simulink model "MSFartoystyring_sine"  (R2015b)
settings: Solver=ode45  StartTime=tstart  StopTime=tstop  RelTol=1e-3
values from neighbouring files (symbols this model uses):
  c = 0    [AnalyseSurgeSpeed.m]    (also in SurgeDynamicsTest.m; SurgeSpeedTest.m; analyse_dynamics.m; analyse_sway_dynamics.m)
  delta_c = deg2rad(delta_list(i))    [analyse_sway_dynamics.m]    (also in msfartoystyring.m = u(1))
  delta_offset = 0.009    [analyse_sway_dynamics.m]
  Ki_u = 0.1    [Speed controller.mat]
  Kp_u = 20    [Speed controller.mat]
  n_c_k = lsqcurvefit(F,1,nc_list,u_list,[],[],optimset('Display','off'))    [AnalyseSpeedCharacteristis.m]    (also in AnalyseSpeedModel.m; Analyse_steadystate.m; Speed controller.mat = 0.976649736616; Speed_characteristics.mat = 0.976649736616)
  n_c_max = 8.9    [AnalyseSpeedCharacteristis.m]    (also in AnalyseSpeedModel.m; AnalyseSurgeSpeed.m; Analyse_steadystate.m; Speed controller.mat)
  n_dot_max = 0.0436332312999    [Speed controller.mat]
  psi0 = 0    [AnalyseSurgeSpeed.m]    (also in SurgeDynamicsTest.m; SurgeSpeedTest.m; analyse_dynamics.m; analyse_sway_dynamics.m)
  r0 = 0    [AnalyseSurgeSpeed.m]    (also in SurgeDynamicsTest.m; SurgeSpeedTest.m; analyse_dynamics.m; analyse_sway_dynamics.m)
  tsamp = 10    [AnalyseSpeedCharacteristis.m]    (also in AnalyseSpeedModel.m; AnalyseSurgeSpeed.m; Analyse_steadystate.m; SurgeDynamicsTest.m)
  v0 = [0.00001 0]'    [AnalyseSurgeSpeed.m]    (also in SurgeDynamicsTest.m = [1e-7 0]'; SurgeSpeedTest.m = [1e-7 0]'; analyse_dynamics.m = [1e-7 0]'; analyse_sway_dynamics.m = [6.63 0]')
  w_u = 0.011    [Speed controller.mat]
undefined symbols (not defined in the file or in its folder): msfartoystyring
undefined symbols (not defined in the file): p0
settings Model: ExtModeAutoUpdateStatusClock=off  Creator=christh  LastModifiedBy=Erik
settings DataIOCC: SaveFormat=Array  SignalLoggingSaveFormat=ModelDataLogs
settings OptimizationCC: ExpressionDepthLimit=2147483647  InitFltsAndDblsToZero=on
settings DebuggingCC: UnderspecifiedInitializationDetection=Classic  MergeDetectMultiDrivingBlocksExec=none  SolverPrmCheckMsg=warning  FcnCallInpInsideContextMsg=UseLocalSettings  StateNameClashWarn=warning
settings HardwareCC: ProdBitPerPointer=32  ProdLargestAtomicFloat=None  ProdIntDivRoundTo=Undefined  ProdEndianess=Unspecified  ProdWordSize=32  ProdHWDeviceType=32-bit Generic
settings GRTTargetCC: GeneratePreprocessorConditionals=Disable all  CombineOutputUpdateFcns=off  GRTInterface=on
settings ConfigComp: CovModelRefEnable=Off

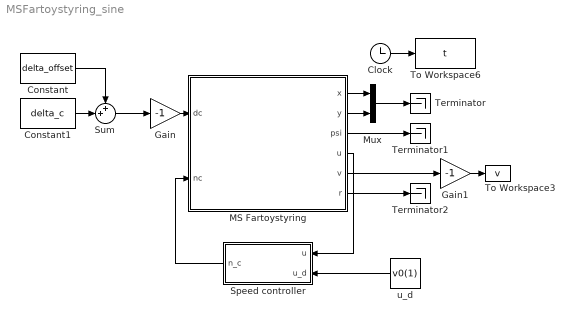
== system MSFartoystyring_sine ==
  Clock : Clock
  Constant : Constant  Value=delta_offset
  Constant1 : Constant  Value=delta_c
  Gain : Gain  Gain=-1
  Gain1 : Gain  Gain=-1
  MS Fartoystyring : Subsystem  mask(MS Fartoystyring for Assignment 3 G&C){x0=p0(1), y0=p0(2), u0=v0(1), v0=v0(2), psi0=psi0, r0=r0, c=c}
      mask prompts: x0 "x(t0) (m)"; y0 "y(t0) (m)"; u0 "u(t0) (m/s)"; v0 "v(t0) (m/s)"; psi0 "psi(t0) (rad)"; r0 "r(t0) (rad/s)"; c "current (0 or 1)"
      mask help:
      | Block corresponding to Figure 1 in the assignment text. Gives the response of the ship.
      |
      | The design speed of MS Fartoystyring is u=8.23 m/s.
      |
      | Input:
      | dc: commanded rudder (rad), dmax=25*pi/180
      | nc: commanded shaft speed (rad/s), nmax=85*2*pi/60
      |
      | Output:
      | x: north pos (m)
      | y: east pos (m)
      | u: surge (m/s)
      | v: sway (m/s)
      | psi: heading (rad)
      | r: yaw (rad/s)
      mask Help: Comments, bugs and help requests can be directed to the TA. Email on course website.
  Mux : Mux  Inputs=2
  Speed controller : Subsystem
  Sum : Sum  Inputs=++|
  Terminator : Terminator
  Terminator1 : Terminator
  Terminator2 : Terminator
  To Workspace3 : ToWorkspace  VariableName=v  SampleTime=tsamp
  To Workspace6 : ToWorkspace  VariableName=t  SampleTime=tsamp
  u_d : Constant  Value=v0(1)
  wires:
  Clock/1 -> To Workspace6/1
  MS Fartoystyring/1(x) -> Mux/1
  MS Fartoystyring/2(y) -> Mux/2
  MS Fartoystyring/4(u) -> Speed controller/1(u)
  MS Fartoystyring/5(v) -> Gain1/1
  Mux/1 -> Terminator/1
  MS Fartoystyring/3(psi) -> Terminator1/1
  MS Fartoystyring/6(r) -> Terminator2/1
  Gain/1 -> MS Fartoystyring/1(dc)
  Constant1/1 -> Sum/2
  Sum/1 -> Gain/1
  Constant/1 -> Sum/1
  Speed controller/1(n_c) -> MS Fartoystyring/2(nc)
  u_d/1 -> Speed controller/2(u_d)
  Gain1/1 -> To Workspace3/1

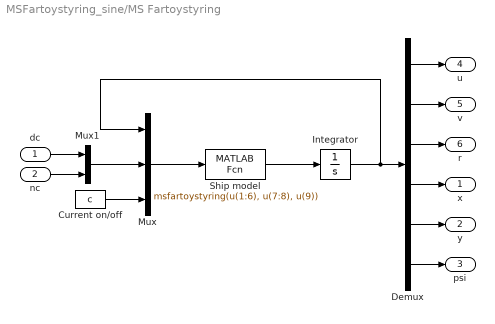
== system MSFartoystyring_sine/MS Fartoystyring ==
  dc : Inport
  nc : Inport  Port=2
  Current on/off : Constant  Value=c
  Demux : Demux  Outputs=6
  Integrator : Integrator  InitialCondition=[u0 v0 r0 x0 y0 psi0]'
  Mux : Mux  Inputs=3
  Mux1 : Mux  Inputs=2
  Ship model : MATLABFcn  MATLABFcn=msfartoystyring(u(1:6), u(7:8), u(9))  OutputDimensions=6
  x : Outport
  y : Outport  Port=2
  psi : Outport  Port=3
  u : Outport  Port=4
  v : Outport  Port=5
  r : Outport  Port=6
  wires:
  Integrator/1 -> Mux/1, Demux/1
  Mux1/1 -> Mux/2
  dc/1 -> Mux1/1
  nc/1 -> Mux1/2
  Demux/1 -> u/1
  Demux/2 -> v/1
  Demux/3 -> r/1
  Demux/4 -> x/1
  Demux/5 -> y/1
  Demux/6 -> psi/1
  Current on/off/1 -> Mux/3
  Ship model/1 -> Integrator/1
  Mux/1 -> Ship model/1

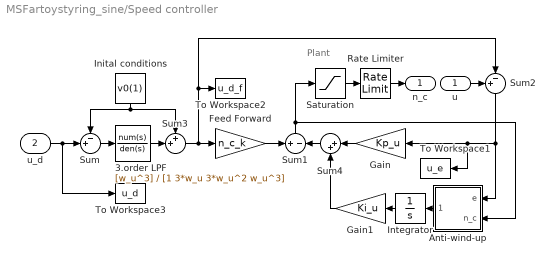
== system MSFartoystyring_sine/Speed controller ==
  note: Plant
  u : Inport
  u_d : Inport  Port=2
  3.order LPF : TransferFcn  Numerator=[w_u^3]  Denominator=[1 3*w_u 3*w_u^2 w_u^3]
  Anti-wind-up : MATLAB Function  TreatAsAtomicUnit=on
  Feed Forward : Gain  Gain=n_c_k
  Gain : Gain  Gain=Kp_u
  Gain1 : Gain  Gain=Ki_u
  Inital conditions : Constant  Value=v0(1)
  Integrator : Integrator
  Rate Limiter : RateLimiter  RisingSlewLimit=n_dot_max  FallingSlewLimit=-n_dot_max
  Saturation : Saturate  UpperLimit=n_c_max  LowerLimit=0.2
  Sum : Sum  Inputs=-+|
  Sum1 : Sum  Inputs=+-
  Sum2 : Sum  Inputs=+-|
  Sum3 : Sum  Inputs=++|
  Sum4 : Sum  Inputs=|++
  To Workspace1 : ToWorkspace  VariableName=u_e  SampleTime=tsamp
  To Workspace2 : ToWorkspace  VariableName=u_d_f  SampleTime=tsamp
  To Workspace3 : ToWorkspace  VariableName=u_d  SampleTime=tsamp
  n_c : Outport
  wires:
  Sum1/1 -> Anti-wind-up/2(n_c), Saturation/1
  Saturation/1 -> Rate Limiter/1
  Rate Limiter/1 -> n_c/1
  u_d/1 -> Sum/2, To Workspace3/1
  Feed Forward/1 -> Sum1/1
  u/1 -> Sum2/1
  Sum2/1 -> To Workspace1/1, Gain/1, Anti-wind-up/1(e)
  Sum/1 -> 3.order LPF/1
  Inital conditions/1 -> Sum/1, Sum3/1
  3.order LPF/1 -> Sum3/2
  Sum3/1 -> Sum2/2, To Workspace2/1, Feed Forward/1
  Integrator/1 -> Gain1/1
  Sum4/1 -> Sum1/2
  Gain/1 -> Sum4/1
  Gain1/1 -> Sum4/2
  Anti-wind-up/1(e_out) -> Integrator/1

== matlab function MSFartoystyring_sine/Speed controller/Anti-wind-up ==
  data: e input; e_out output; n_c input
function e_out = fcn(e, n_c)
    n_c_max = 8.9; 
    if n_c >= n_c_max
        e_out = 0;
    else
        e_out = e;
    end
end
